simulink model "control_motor_test"  (R2013b)
settings: Solver=ode3  SolverMode=SingleTasking  StartTime=0.0  StopTime=5  RelTol=1e-3
libraries: legonxtlib x4
settings Model: ExtModeTrigDuration=2  Creator=Alphonso Monk  LastModifiedBy=Alphonso Monk
settings DataIOCC: SignalLoggingSaveFormat=ModelDataLogs
settings OptimizationCC: OptimizeModelRefInitCode=on  LifeSpan=1
settings DebuggingCC: SolverPrmCheckMsg=none  StateNameClashWarn=warning
settings HardwareCC: ProdLargestAtomicInteger=Long  ProdLargestAtomicFloat=Float  ProdEndianess=LittleEndian  ProdHWDeviceType=ARM Compatible->ARM 7
settings RTWCC: SystemTargetFile=realtime.tlc  GenerateMakefile=off  TemplateMakefile=realtime.tmf  Description=Run on Target Hardware  RTWVerbose=off  ProcessScript=realtime_make_rtw_hook
settings STFCustomTargetCC: TargetLibSuffix=.a  GenerateSampleERTMain=on  ERTCustomFileBanners=on  SupportNonInlinedSFcns=off  SupportVariableSizeSignals=on  MATLABClassNameForMDSCustomization=Simulink.SoftwareTarget.ERTCustomization  GRTInterface=off  SystemTargetFile=realtime.tlc
settings ERTTargetCC: CodeReplacementLibrary=ANSI_C  GenerateSampleERTMain=on  ParMdlRefBuildCompliant=off  CompOptLevelCompliant=off  ConcurrentExecutionCompliant=off  CombineOutputUpdateFcns=off  ERTFirstTimeCompliant=off  SupportContinuousTime=on  SupportVariableSizeSignals=on  ModelStepFunctionPrototypeControlCompliant=off  CPPClassGenCompliant=off  ExtModeTransport=2  ExtModeMexFile=ext_serial_win32_comm_no_acks_rtt  ExtModeMexArgs=0 1 9600  InlinedParameterPlacement=NonHierarchical  ERTSrcFileBannerTemplate=realtime_code_template.cgt  ERTHdrFileBannerTemplate=realtime_code_template.cgt  ERTDataSrcFileTemplate=realtime_code_template.cgt  ERTDataHdrFileTemplate=realtime_code_template.cgt  ERTCustomFileTemplate=realtime_file_process.tlc

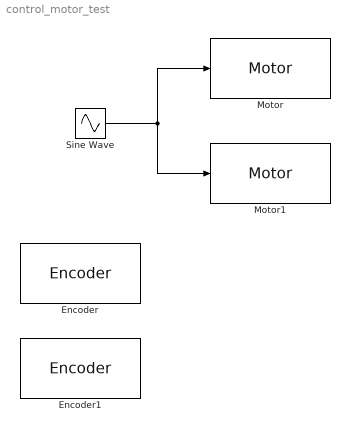
== system control_motor_test ==
  Encoder : legonxtlib/Encoder  portNumber=B  opMode=No reset  sampleTime=0.1
  Encoder1 : legonxtlib/Encoder  portNumber=A  opMode=No reset  sampleTime=0.1
  Motor : legonxtlib/Motor  sportNumber=B  sstopAction=Brake
  Motor1 : legonxtlib/Motor  sportNumber=C  sstopAction=Brake
  Sine Wave : Sin  Amplitude=100  Frequency=5  SampleTime=0
  wires:
  Sine Wave/1 -> Motor/1, Motor1/1
